simulink model "simulator"  (R2024b)
settings: Solver=VariableStepAuto  StartTime=0  StopTime=30  FixedStep=Ts  MinStep=1e-5
undefined symbols (not defined in the file or in its folder): x0
settings Model: SimulationMode=accelerator  Creator=bduprey  LastModifiedBy=kseki
settings DataIOCC: SaveFormat=Array  SaveOutput=off  SignalLogging=off  DSMLogging=off  SaveTime=off
settings OptimizationCC: BlockReduction=off  BooleanDataType=off  ReuseModelBlockBuffer=off  ExpressionDepthLimit=2147483647  LifeSpan=inf
settings DebuggingCC: SaveWithParameterizedLinksMsg=none  MergeDetectMultiDrivingBlocksExec=none  SignalResolutionControl=TryResolveAllWithWarning  MultiTaskDSMMsg=warning  MultiTaskCondExecSysMsg=none  UnconnectedInputMsg=warning  UnconnectedOutputMsg=warning  UnconnectedLineMsg=warning  StateNameClashWarn=warning  SFUnexpectedBacktrackingDiag=warning  SFNoUnconditionalDefaultTransitionDiag=warning  SFExecutionAtInitializationDiag=none  UnderSpecifiedDimensionMsg=warning  ArithmeticOperatorsInVariantConditions=warning
settings HardwareCC: ProdBitPerPointer=32  ProdBitPerSizeT=32  ProdBitPerPtrDiffT=32  ProdLargestAtomicFloat=None  ProdIntDivRoundTo=Undefined  ProdEndianess=Unspecified  ProdWordSize=32  ProdHWDeviceType=32-bit Generic  TargetUnknown=on
settings ModelReferenceCC: EnableRefExpFcnMdlSchedulingChecks=on  PropagateSignalLabelsOutOfModel=off
settings SFSimCC: SimUseLocalCustomCode=off  CustomCodeUndefinedFunction=UseInterfaceOnly
settings RTWCC: TemplateMakefile=grt_vc.tmf  RTWUseLocalCustomCode=off  GPUComputeCapability=3.5  DLArmComputeVersion=19.05
settings CodeAppCC: StateflowObjectComments=on
settings GRTTargetCC: TargetFcnLib=ansi_tfl_tmw.mat  TargetLangStandard=C89/C90 (ANSI)  CombineOutputUpdateFcns=off  GRTInterface=on
settings ConfigComp: CovMetricSettings=dw  CovSaveCumulativeToWorkspaceVar=on  CovSaveSingleToWorkspaceVar=on  CovExternalEMLEnable=off

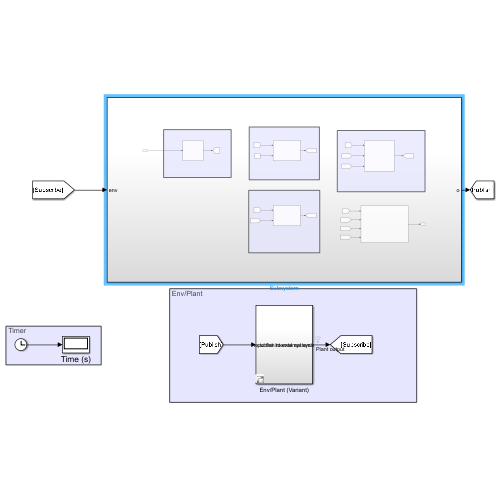
[thumbnail: Simulink's stored preview of the top-level diagram]
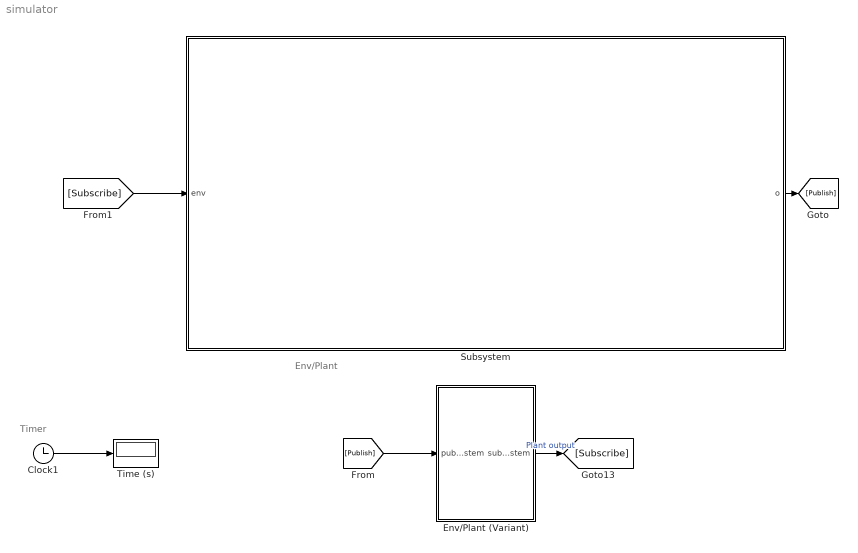
== system simulator ==
  note: Env/Plant
  note: Timer
  Clock1 : Clock
  Env/Plant (Variant) : Subsystem  Variant=on  AllowZeroVariantControls=on  PropagateVariantConditions=on
  Subsystem : Subsystem
  Time (s) : Display
      settings: Format=bank  Decimation=100
  wires:
  Clock1/1 -> Time (s)/1
  Env/Plant (Variant)/1(subscribe to the internal system) -> [Subscribe]  "Plant output"
  Subsystem/1(o) -> [Publish]
  [Publish] -> Env/Plant (Variant)/1(publish to external system)
  [Subscribe] -> Subsystem/1(env)

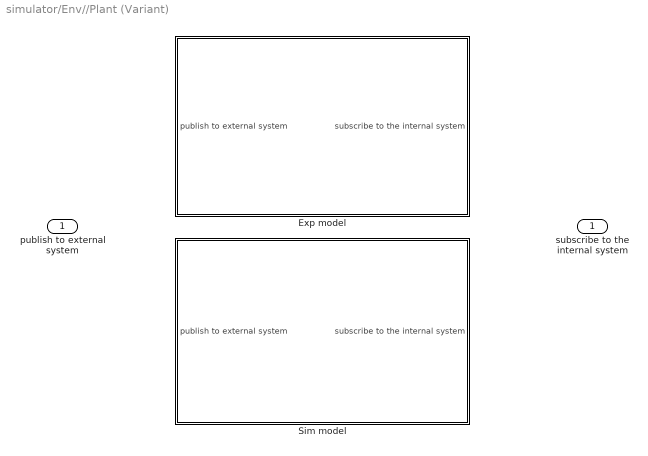
== system simulator/Env//Plant (Variant) ==
  publish to external system : Inport
  Exp model : Subsystem  VariantControl="Flag.Model.Type == \"TruckSim\""
  Sim model : Subsystem  VariantControl="Flag.Model.Type == \"ThreeDoF\""
  subscribe to the internal system : Outport

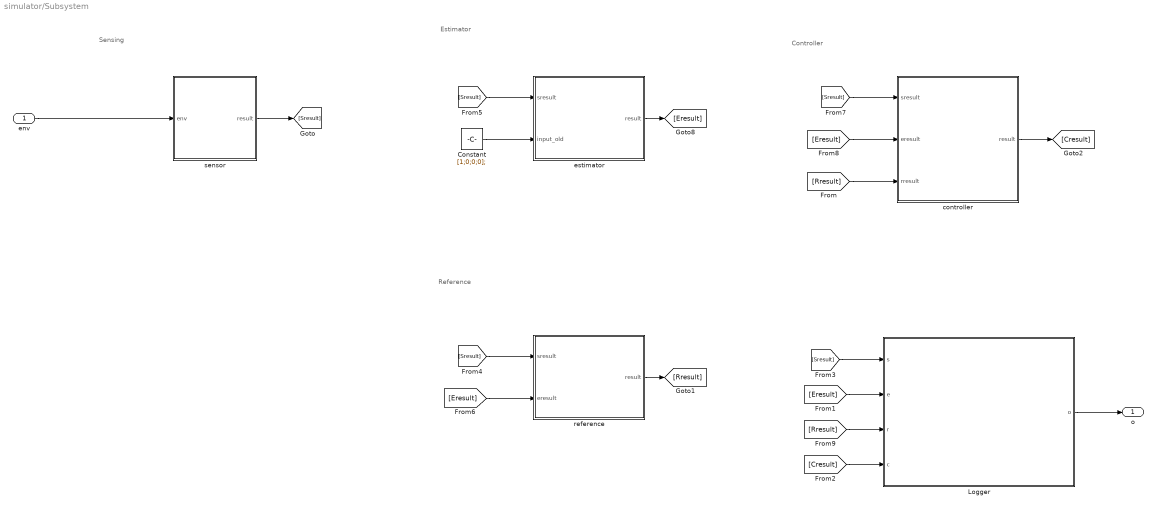
== system simulator/Subsystem ==
  note: Sensing
  note: Reference
  note: Controller
  note: Estimator
  env : Inport
  Constant : Constant  Value=[1;0;0;0];
  Logger : MATLAB Function  TreatAsAtomicUnit=on
  controller : MATLAB Function  TreatAsAtomicUnit=on
  estimator : MATLAB Function  TreatAsAtomicUnit=on
  reference : MATLAB Function  TreatAsAtomicUnit=on
  sensor : MATLAB Function  TreatAsAtomicUnit=on
  o : Outport
  wires:
  estimator/1(result) -> [Eresult]
  Constant/1 -> estimator/2(input_old)
  [Sresult] -> estimator/1(sresult)
  env/1 -> sensor/1(env)
  sensor/1(result) -> [Sresult]
  [Sresult] -> Logger/1(s)
  reference/1(result) -> [Rresult]
  [Sresult] -> reference/1(sresult)
  [Eresult] -> reference/2(eresult)
  [Eresult] -> controller/2(eresult)
  [Sresult] -> controller/1(sresult)
  controller/1(result) -> [Cresult]
  [Rresult] -> controller/3(rresult)
  [Eresult] -> Logger/2(e)
  [Rresult] -> Logger/3(r)
  [Cresult] -> Logger/4(c)
  Logger/1(o) -> o/1

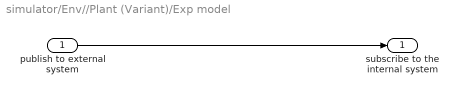
== system simulator/Env//Plant (Variant)/Exp model ==
  publish to external system : Inport
  subscribe to the internal system : Outport
  wires:
  publish to external system/1 -> subscribe to the internal system/1

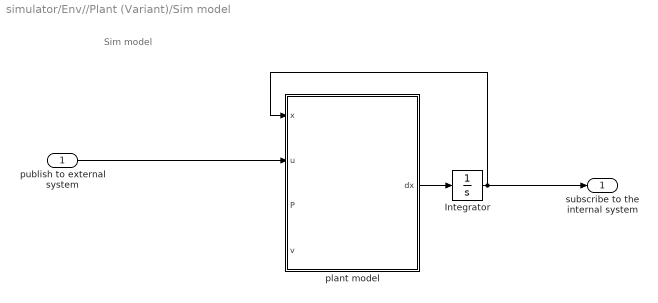
== system simulator/Env//Plant (Variant)/Sim model ==
  note: Sim model
  publish to external system : Inport
  Integrator : Integrator  InitialCondition=x0
  plant model : MATLAB Function  TreatAsAtomicUnit=on
  subscribe to the internal system : Outport
  wires:
  plant model/1(dx) -> Integrator/1
  publish to external system/1 -> plant model/2(u)
  Integrator/1 -> plant model/1(x), subscribe to the internal system/1

== matlab function simulator/Subsystem/estimator ==
  data: sresult input; result output; input_old input
function result = Estimator_simulink(sresult,input_old)
result = agent.estimator.do(sresult,input_old);

== matlab function simulator/Subsystem/Logger ==
  data: s input; o output; e input; r input; c input
function o = logger_simulink(s,e,r,c)

o = logger.loggin(s,e,r,c);

== matlab function simulator/Subsystem/sensor ==
  data: env input; result output
function result = Sensor_simulink(env)
result = agent.sensor.do(env);

== matlab function simulator/Subsystem/reference ==
  data: sresult input; result output; eresult input
function result = Reference_simulink(sresult,eresult)
result = agent.reference.do(sresult,eresult);

== matlab function simulator/Subsystem/controller ==
  data: sresult input; result output; eresult input; rresult input
function result = Controller_simulink(sresult,eresult,rresult)
result = agent.controller.do(sresult,eresult,rresult);

== matlab function simulator/Env//Plant (Variant)/Sim model/plant model ==
  data: x input; dx output; u input; P input; v input
function dx  = plant_model(x,u, P, v)
% continuous time plant model
% [input]
% x  : state
% u  : input
% P  : parameter
% v  : disturbance

% [output]
% dx : dx/dt
dx = plant_c(x(:),u(:),P(:))+v(:);
